simulink model "cordicq2_14"  (R2024b)
settings: Solver=VariableStepAuto  StartTime=0.0  StopTime=4e-6  RelTol=1e-3
libraries: fillib x1
settings Model: Creator=ETLCLab-Tesisti  LastModifiedBy=ETLCLab-Tesisti

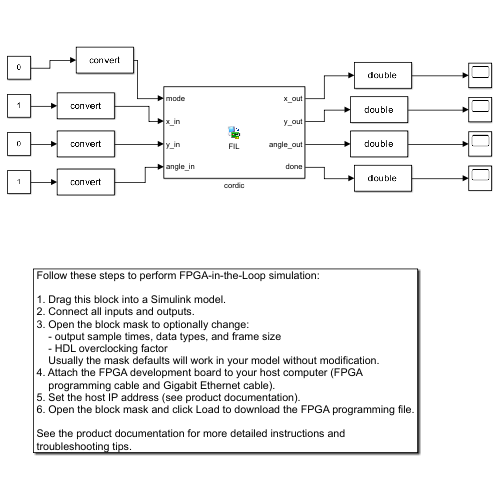
[thumbnail: Simulink's stored preview of the top-level diagram]
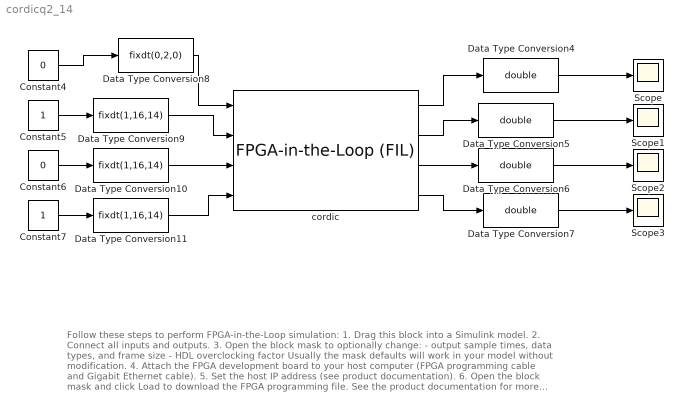
== system cordicq2_14 ==
  note: Follow these steps to perform FPGA-in-the-Loop simulation:
      |
      | 1. Drag this block into a Simulink model.
      | 2. Connect all inputs and outputs.
      | 3. Open the block mask to optionally change:
      |     - output sample times, data types, and frame size
      |     - HDL overclocking factor
      |     Usually the mask defaults will work in your model without modification.
      | 4. Attach the FPGA development board to your host computer (FPGA
      |     programming cable and Gigabit Ethernet cable).
      | 5. Set the host IP address (see product documentation).
      | 6. Open the block mask and click Load to download the FPGA programming file.
      |
      | See the product documentation for more detailed instructions and
      | troubleshooting tips.
  Constant4 : Constant  Value=0  OutDataTypeStr=double  SampleTime=1/25e6
  Constant5 : Constant  SampleTime=1/25e6
  Constant6 : Constant  Value=0  SampleTime=1/25e6
  Constant7 : Constant  SampleTime=1/25e6
  Data Type Conversion10 : DataTypeConversion  OutDataTypeStr=fixdt(1,16,14)  RndMeth=Floor
  Data Type Conversion11 : DataTypeConversion  OutDataTypeStr=fixdt(1,16,14)  RndMeth=Floor
  Data Type Conversion{4..7} (4 alike) : DataTypeConversion  OutDataTypeStr=double  RndMeth=Floor
  Data Type Conversion8 : DataTypeConversion  OutDataTypeStr=fixdt(0,2,0)  RndMeth=Floor
  Data Type Conversion9 : DataTypeConversion  OutDataTypeStr=fixdt(1,16,14)  RndMeth=Floor
  Scope{,1..3} (4 alike) : Scope
  cordic : fillib/FPGA-in-the-Loop (FIL)  ForceInterfaceUpdate=0.14189
  wires:
  Data Type Conversion8/1 -> cordic/1
  Data Type Conversion10/1 -> cordic/3
  Data Type Conversion11/1 -> cordic/4
  Data Type Conversion9/1 -> cordic/2
  Constant6/1 -> Data Type Conversion10/1
  Constant4/1 -> Data Type Conversion8/1
  Constant5/1 -> Data Type Conversion9/1
  Constant7/1 -> Data Type Conversion11/1
  cordic/4 -> Data Type Conversion7/1
  cordic/1 -> Data Type Conversion4/1
  cordic/3 -> Data Type Conversion6/1
  Data Type Conversion6/1 -> Scope2/1
  Data Type Conversion4/1 -> Scope/1
  cordic/2 -> Data Type Conversion5/1
  Data Type Conversion5/1 -> Scope1/1
  Data Type Conversion7/1 -> Scope3/1
